simulink model "Longitudinal_model"  (R2018b)
settings: Solver=ode4  StartTime=0.0  StopTime=30  FixedStep=0.001  RelTol=1e-3
values from neighbouring files (symbols this model uses):
  brake_force = 0    [Dinamic_model.m]
  Cf2 = 1    [Dinamic_model.m]
  Cf3 = 1    [Dinamic_model.m]
  Cf4 = 1    [Dinamic_model.m]
  Drag_force_constant = 0.5 * Ro * A * Cd    (= 2.788272)    [Dinamic_model.m]
  Fs = m * g * sin(thetarad)    [Dinamic_model.m]
  Fz1 = Fz / 4    (= 1863.9)    [Dinamic_model.m]
  Fz2 = Fz / 4    (= 1863.9)    [Dinamic_model.m]
  Fz3 = Fz / 4    (= 1863.9)    [Dinamic_model.m]
  Fz4 = Fz / 4    (= 1863.9)    [Dinamic_model.m]
  J1 = 0.9    [Dinamic_model.m]
  J2 = 0.9    [Dinamic_model.m]
  J3 = 0.9    [Dinamic_model.m]
  J4 = 0.9    [Dinamic_model.m]
  m = Fz / g    (= 760)    [Dinamic_model.m]
  r1 = 0.51    [Dinamic_model.m]
  r2 = 0.51    [Dinamic_model.m]
  r3 = 0.51    [Dinamic_model.m]
  r4 = 0.51    [Dinamic_model.m]
  Rx = Cr * m * g * cos(thetarad)    [Dinamic_model.m]
  torque = 1000    [Dinamic_model.m]
undefined symbols (not defined in the file or in its folder): Cf1
settings Model: Creator=Misi  LastModifiedBy=Misi

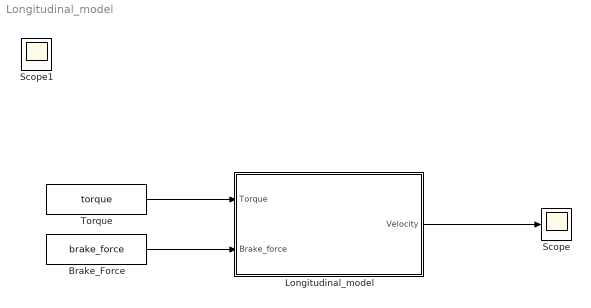
== system Longitudinal_model ==
  Brake_Force : Constant  Value=brake_force
  Longitudinal_model : Subsystem
  Scope : Scope
  Torque : Constant  Value=torque
  Scope1 : Scope
  wires:
  Longitudinal_model/1("Velocity ") -> Scope/1
  Torque/1 -> Longitudinal_model/1("Torque ")
  Brake_Force/1 -> Longitudinal_model/2("Brake_force ")

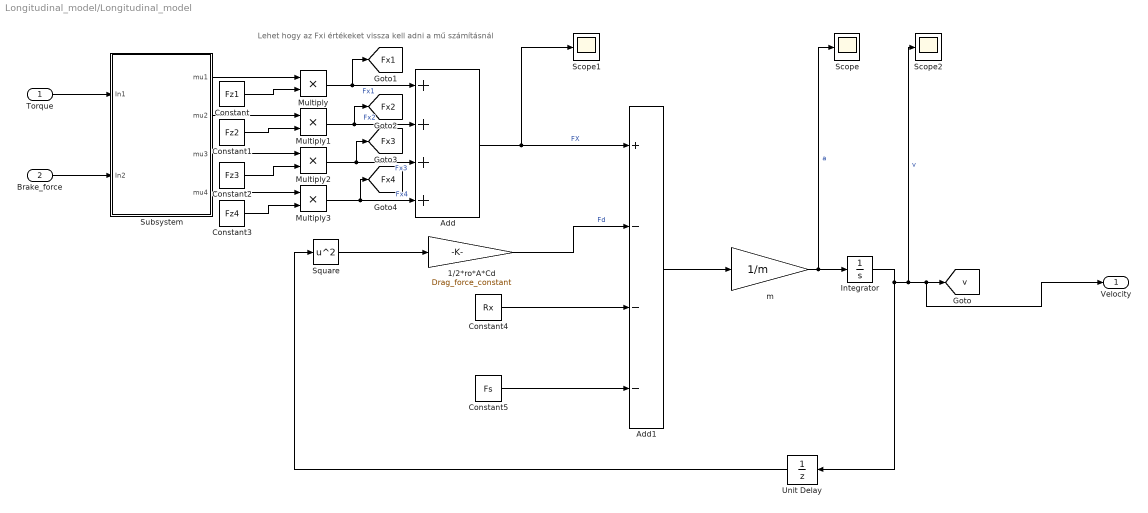
== system Longitudinal_model/Longitudinal_model ==
  note: Lehet hogy az Fxi értékeket vissza kell adni a mű számításnál
  "Torque " : Inport
  "Brake_force " : Inport  Port=2
  1/2*ro*A*Cd : Gain  Gain=Drag_force_constant
  Add : Sum  Inputs=++++
  Add1 : Sum  Inputs=+---
  Constant : Constant  Value=Fz1
  Constant1 : Constant  Value=Fz2
  Constant2 : Constant  Value=Fz3
  Constant3 : Constant  Value=Fz4
  Constant4 : Constant  Value=Rx
  Constant5 : Constant  Value=Fs
  Integrator : Integrator
  Multiply{,1..3} (4 alike) : Product
  Scope : Scope
  Scope1 : Scope
  Scope2 : Scope
  Square : Math  Operator=square  SaturateOnIntegerOverflow=on
  Subsystem : Subsystem
  Unit Delay : UnitDelay  InitialCondition=100  SampleTime=-1
  m : Gain  Gain=1/m
  "Velocity " : Outport
  tag scope: Fx1=global, Fx2=global, Fx3=global, Fx4=global, v=global
  wires:
  "Torque "/1 -> Subsystem/1(In1)
  "Brake_force "/1 -> Subsystem/2(In2)
  Subsystem/1(mu1) -> Multiply/1
  Multiply/1 -> [Fx1], Add/1  "Fx1"
  Multiply1/1 -> [Fx2], Add/2  "Fx2"
  Multiply2/1 -> [Fx3], Add/3  "Fx3"
  Multiply3/1 -> [Fx4], Add/4  "Fx4"
  Add/1 -> Scope1/1, Add1/1  "FX"
  Square/1 -> 1/2*ro*A*Cd/1
  1/2*ro*A*Cd/1 -> Add1/2  "Fd"
  Add1/1 -> m/1
  m/1 -> Scope/1, Integrator/1  "a"
  Integrator/1 -> Unit Delay/1, Scope2/1, "Velocity "/1, [v]  "v"
  Unit Delay/1 -> Square/1
  Constant/1 -> Multiply/2
  Constant1/1 -> Multiply1/2
  Subsystem/2(mu2) -> Multiply1/1
  Constant2/1 -> Multiply2/2
  Constant3/1 -> Multiply3/2
  Subsystem/4(mu4) -> Multiply3/1
  Subsystem/3(mu3) -> Multiply2/1
  Constant4/1 -> Add1/3
  Constant5/1 -> Add1/4

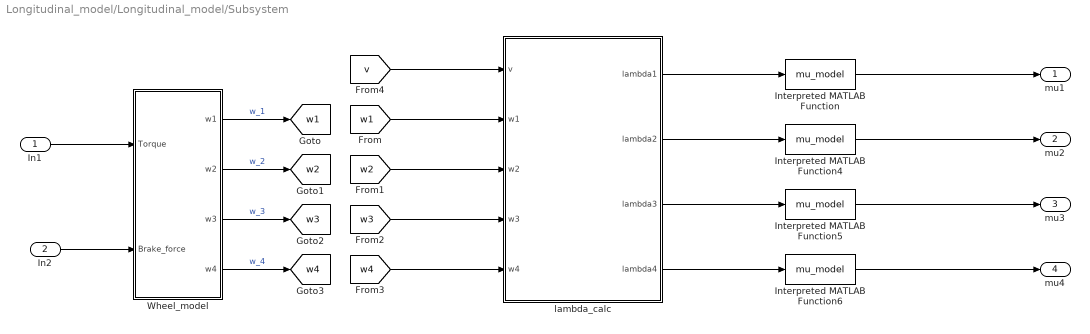
== system Longitudinal_model/Longitudinal_model/Subsystem ==
  In1 : Inport
  In2 : Inport  Port=2
  Interpreted MATLAB Function{,4..6} (4 alike) : MATLABFcn  MATLABFcn=mu_model  OutputDimensions=4
  "Wheel_model " : Subsystem
  lambda_calc : Subsystem
  mu1 : Outport
  mu2 : Outport  Port=2
  mu3 : Outport  Port=3
  mu4 : Outport  Port=4
  tag scope: w1=global, w2=global, w3=global, w4=global
  wires:
  [w4] -> lambda_calc/5(w4)
  "Wheel_model "/1(w1) -> [w1]  "w_1"
  In2/1 -> "Wheel_model "/2(Brake_force)
  [w3] -> lambda_calc/4(w3)
  [w1] -> lambda_calc/2(w1)
  [w2] -> lambda_calc/3(w2)
  "Wheel_model "/4("w4 ") -> [w4]  "w_4"
  "Wheel_model "/3(w3) -> [w3]  "w_3"
  "Wheel_model "/2(w2) -> [w2]  "w_2"
  In1/1 -> "Wheel_model "/1(Torque)
  [v] -> lambda_calc/1(v)
  Interpreted MATLAB Function/1 -> mu1/1
  Interpreted MATLAB Function4/1 -> mu2/1
  Interpreted MATLAB Function5/1 -> mu3/1
  Interpreted MATLAB Function6/1 -> mu4/1
  lambda_calc/1("lambda1 ") -> Interpreted MATLAB Function/1
  lambda_calc/2(lambda2) -> Interpreted MATLAB Function4/1
  lambda_calc/3(lambda3) -> Interpreted MATLAB Function5/1
  lambda_calc/4(lambda4) -> Interpreted MATLAB Function6/1

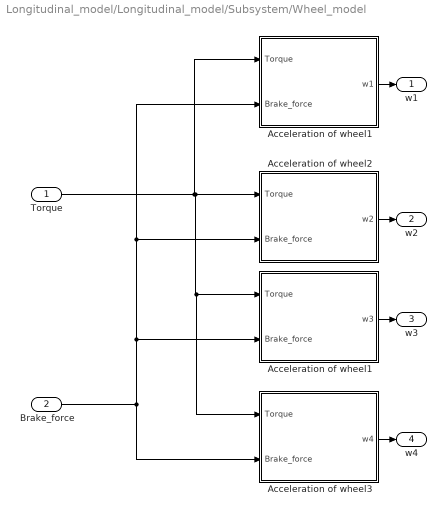
== system Longitudinal_model/Longitudinal_model/Subsystem/Wheel_model  ==
  Torque : Inport
  Brake_force : Inport  Port=2
  Acceleration of wheel1 : Subsystem
  "Acceleration of wheel1 " : Subsystem
  Acceleration of wheel2 : Subsystem
  Acceleration of wheel3 : Subsystem
  w1 : Outport
  w2 : Outport  Port=2
  w3 : Outport  Port=3
  "w4 " : Outport  Port=4
  wires:
  Brake_force/1 -> Acceleration of wheel3/2("Brake_force "), Acceleration of wheel1/2("Brake_force "), Acceleration of wheel2/2("Brake_force "), "Acceleration of wheel1 "/2("Brake_force ")
  Torque/1 -> Acceleration of wheel2/1("Torque "), Acceleration of wheel3/1("Torque "), Acceleration of wheel1/1("Torque "), "Acceleration of wheel1 "/1("Torque ")
  Acceleration of wheel2/1("w2 ") -> w2/1
  "Acceleration of wheel1 "/1("w1 ") -> w1/1
  Acceleration of wheel1/1("w3 ") -> w3/1
  Acceleration of wheel3/1("w4 ") -> "w4 "/1

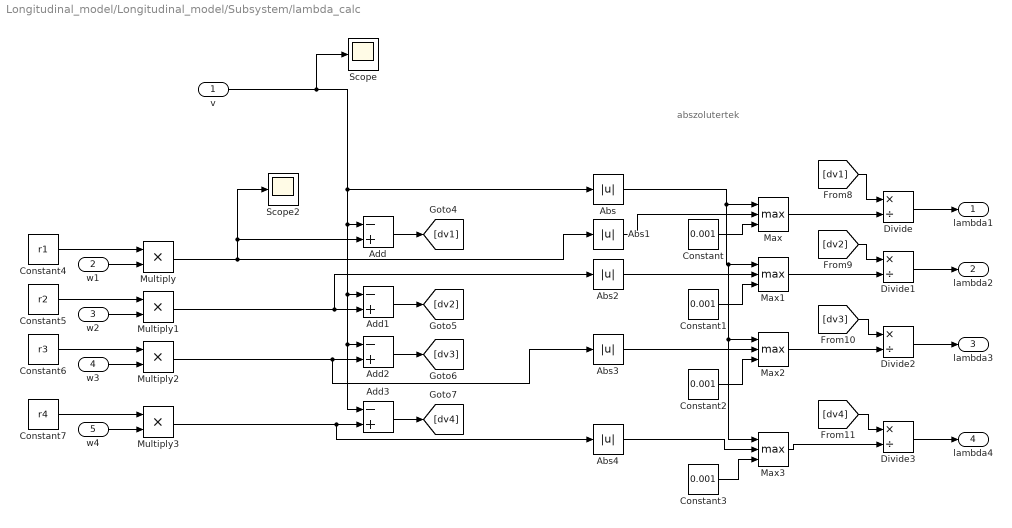
== system Longitudinal_model/Longitudinal_model/Subsystem/lambda_calc ==
  note: abszolutertek
  v : Inport
  w1 : Inport  Port=2
  w2 : Inport  Port=3
  w3 : Inport  Port=4
  w4 : Inport  Port=5
  Abs{,1..4} (5 alike) : Abs
  Add{,1..3} (4 alike) : Sum  Inputs=-+
  Constant{,1..3} (4 alike) : Constant  Value=0.001
  Constant4 : Constant  Value=r1
  Constant5 : Constant  Value=r2
  Constant6 : Constant  Value=r3
  Constant7 : Constant  Value=r4
  Divide{,1..3} (4 alike) : Product  Inputs=*/
  Max{,1..3} (4 alike) : MinMax  Function=max  Inputs=3
  Multiply{,1..3} (4 alike) : Product
  Scope : Scope
  Scope2 : Scope
  "lambda1 " : Outport
  lambda2 : Outport  Port=2
  lambda3 : Outport  Port=3
  lambda4 : Outport  Port=4
  wires:
  [dv2] -> Divide1/1
  Add3/1 -> [dv4]
  Max2/1 -> Divide2/2
  Max1/1 -> Divide1/2
  [dv1] -> Divide/1
  Add/1 -> [dv1]
  v/1 -> Scope/1, Abs/1, Add3/1, Add2/1, Add1/1, Add/1
  w4/1 -> Multiply3/2
  Constant4/1 -> Multiply/1
  Divide3/1 -> lambda4/1
  [dv4] -> Divide3/1
  Max/1 -> Divide/2
  Multiply2/1 -> Abs3/1, Add2/2
  Multiply3/1 -> Abs4/1, Add3/2
  Max3/1 -> Divide3/2
  Divide1/1 -> lambda2/1
  [dv3] -> Divide2/1
  Add2/1 -> [dv3]
  Multiply1/1 -> Abs2/1, Add1/2
  w1/1 -> Multiply/2
  w2/1 -> Multiply1/2
  Add1/1 -> [dv2]
  w3/1 -> Multiply2/2
  Divide/1 -> "lambda1 "/1
  Divide2/1 -> lambda3/1
  Constant5/1 -> Multiply1/1
  Constant6/1 -> Multiply2/1
  Constant7/1 -> Multiply3/1
  Constant1/1 -> Max1/3
  Constant/1 -> Max/3
  Constant2/1 -> Max2/3
  Constant3/1 -> Max3/3
  Multiply/1 -> Abs1/1, Scope2/1, Add/2
  Abs/1 -> Max3/1, Max2/1, Max1/1, Max/1
  Abs1/1 -> Max/2
  Abs2/1 -> Max1/2
  Abs3/1 -> Max2/2
  Abs4/1 -> Max3/2

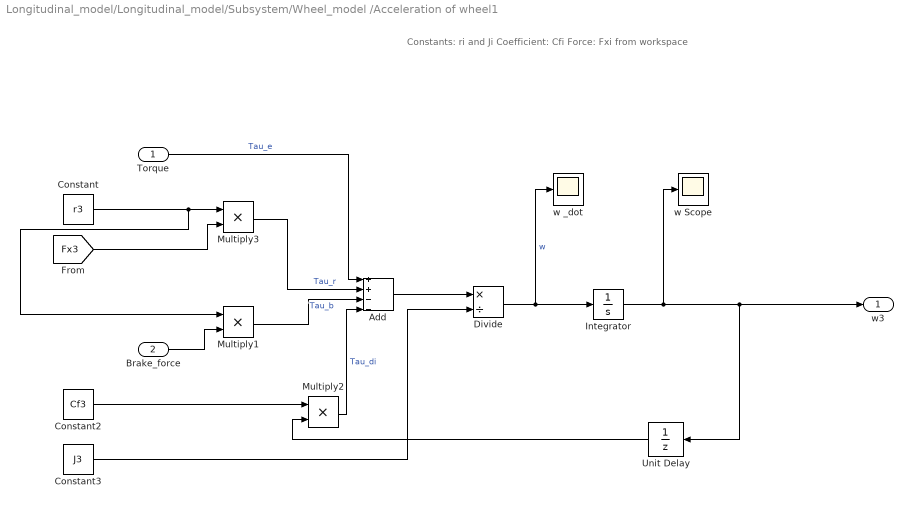
== system Longitudinal_model/Longitudinal_model/Subsystem/Wheel_model /Acceleration of wheel1 ==
  note: Constants: ri and Ji
      | Coefficient: Cfi
      | Force: Fxi
      | from workspace
  "Torque " : Inport
  "Brake_force " : Inport  Port=2
  Add : Sum  Inputs=++--
  Constant : Constant  Value=r3
  Constant2 : Constant  Value=Cf3
  Constant3 : Constant  Value=J3
  Divide : Product  Inputs=*/
  Integrator : Integrator
  Multiply1 : Product
  Multiply2 : Product
  Multiply3 : Product
  Unit Delay : UnitDelay  SampleTime=-1
  w Scope : Scope
  "w _dot " : Scope
  "w3 " : Outport
  wires:
  Multiply2/1 -> Add/4  "Tau_di"
  Divide/1 -> "w _dot "/1, Integrator/1  "w"
  Constant2/1 -> Multiply2/1
  Multiply1/1 -> Add/3  "Tau_b"
  "Brake_force "/1 -> Multiply1/2
  "Torque "/1 -> Add/1  "Tau_e"
  Constant/1 -> Multiply1/1, Multiply3/1
  [Fx3] -> Multiply3/2
  Multiply3/1 -> Add/2  "Tau_r"
  Add/1 -> Divide/1
  Integrator/1 -> "w3 "/1, Unit Delay/1, w Scope/1
  Unit Delay/1 -> Multiply2/2
  Constant3/1 -> Divide/2

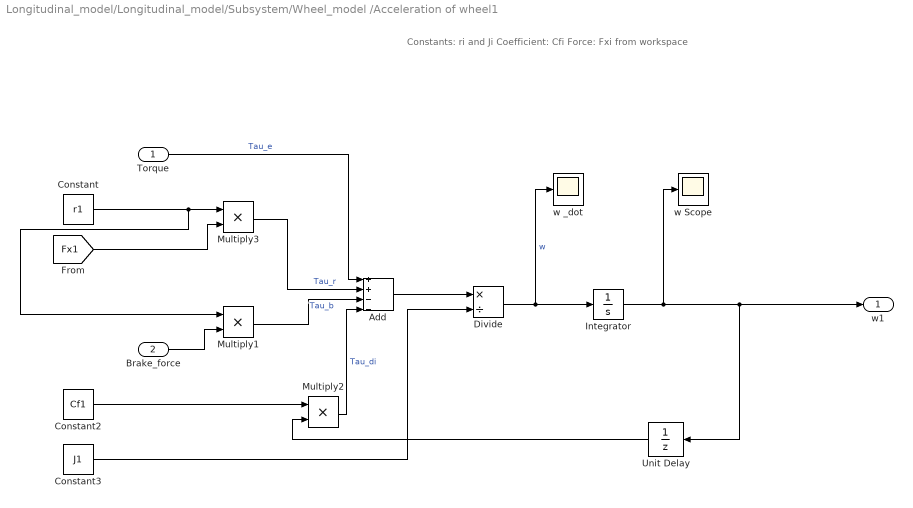
== system Longitudinal_model/Longitudinal_model/Subsystem/Wheel_model /Acceleration of wheel1  ==
  note: Constants: ri and Ji
      | Coefficient: Cfi
      | Force: Fxi
      | from workspace
  "Torque " : Inport
  "Brake_force " : Inport  Port=2
  Add : Sum  Inputs=++--
  Constant : Constant  Value=r1
  Constant2 : Constant  Value=Cf1
  Constant3 : Constant  Value=J1
  Divide : Product  Inputs=*/
  Integrator : Integrator
  Multiply1 : Product
  Multiply2 : Product
  Multiply3 : Product
  Unit Delay : UnitDelay  SampleTime=-1
  w Scope : Scope
  "w _dot " : Scope
  "w1 " : Outport
  wires:
  Multiply2/1 -> Add/4  "Tau_di"
  Divide/1 -> "w _dot "/1, Integrator/1  "w"
  Constant2/1 -> Multiply2/1
  Multiply1/1 -> Add/3  "Tau_b"
  "Brake_force "/1 -> Multiply1/2
  "Torque "/1 -> Add/1  "Tau_e"
  Constant/1 -> Multiply1/1, Multiply3/1
  [Fx1] -> Multiply3/2
  Multiply3/1 -> Add/2  "Tau_r"
  Add/1 -> Divide/1
  Integrator/1 -> "w1 "/1, Unit Delay/1, w Scope/1
  Unit Delay/1 -> Multiply2/2
  Constant3/1 -> Divide/2

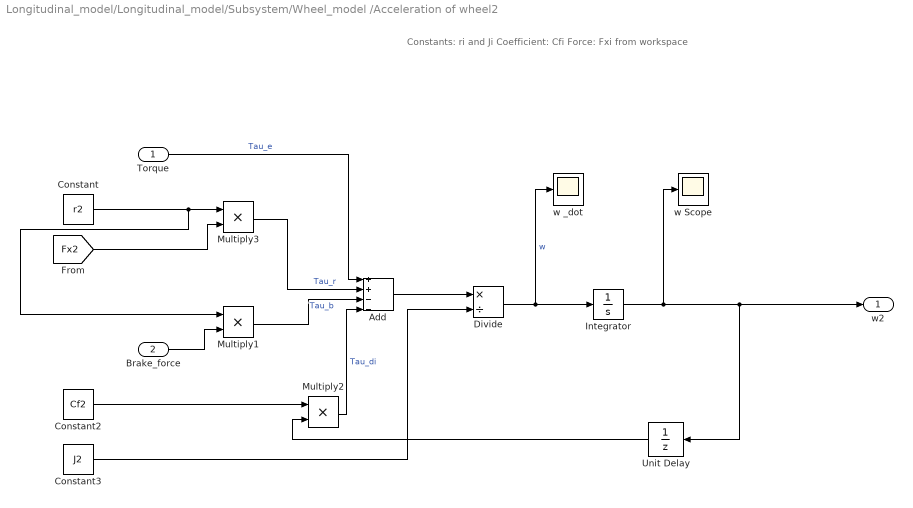
== system Longitudinal_model/Longitudinal_model/Subsystem/Wheel_model /Acceleration of wheel2 ==
  note: Constants: ri and Ji
      | Coefficient: Cfi
      | Force: Fxi
      | from workspace
  "Torque " : Inport
  "Brake_force " : Inport  Port=2
  Add : Sum  Inputs=++--
  Constant : Constant  Value=r2
  Constant2 : Constant  Value=Cf2
  Constant3 : Constant  Value=J2
  Divide : Product  Inputs=*/
  Integrator : Integrator
  Multiply1 : Product
  Multiply2 : Product
  Multiply3 : Product
  Unit Delay : UnitDelay  SampleTime=-1
  w Scope : Scope
  "w _dot " : Scope
  "w2 " : Outport
  wires:
  Constant3/1 -> Divide/2
  Unit Delay/1 -> Multiply2/2
  Integrator/1 -> w Scope/1, Unit Delay/1, "w2 "/1
  Add/1 -> Divide/1
  Multiply3/1 -> Add/2  "Tau_r"
  [Fx2] -> Multiply3/2
  Constant/1 -> Multiply3/1, Multiply1/1
  "Torque "/1 -> Add/1  "Tau_e"
  "Brake_force "/1 -> Multiply1/2
  Multiply1/1 -> Add/3  "Tau_b"
  Constant2/1 -> Multiply2/1
  Divide/1 -> Integrator/1, "w _dot "/1  "w"
  Multiply2/1 -> Add/4  "Tau_di"

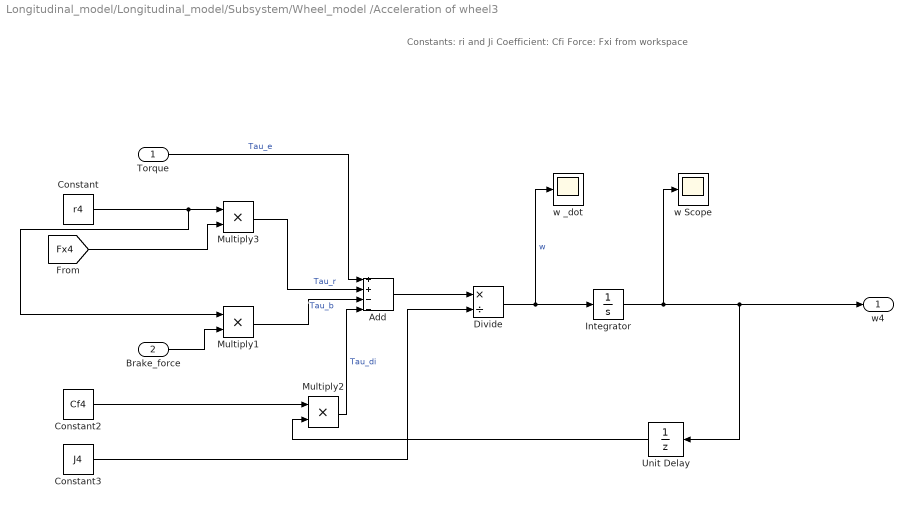
== system Longitudinal_model/Longitudinal_model/Subsystem/Wheel_model /Acceleration of wheel3 ==
  note: Constants: ri and Ji
      | Coefficient: Cfi
      | Force: Fxi
      | from workspace
  "Torque " : Inport
  "Brake_force " : Inport  Port=2
  Add : Sum  Inputs=++--
  Constant : Constant  Value=r4
  Constant2 : Constant  Value=Cf4
  Constant3 : Constant  Value=J4
  Divide : Product  Inputs=*/
  Integrator : Integrator
  Multiply1 : Product
  Multiply2 : Product
  Multiply3 : Product
  Unit Delay : UnitDelay  SampleTime=-1
  w Scope : Scope
  "w _dot " : Scope
  "w4 " : Outport
  wires:
  Constant3/1 -> Divide/2
  Unit Delay/1 -> Multiply2/2
  Integrator/1 -> w Scope/1, Unit Delay/1, "w4 "/1
  Add/1 -> Divide/1
  Multiply3/1 -> Add/2  "Tau_r"
  [Fx4] -> Multiply3/2
  Constant/1 -> Multiply3/1, Multiply1/1
  "Torque "/1 -> Add/1  "Tau_e"
  "Brake_force "/1 -> Multiply1/2
  Multiply1/1 -> Add/3  "Tau_b"
  Constant2/1 -> Multiply2/1
  Divide/1 -> Integrator/1, "w _dot "/1  "w"
  Multiply2/1 -> Add/4  "Tau_di"
